simulink model "RLS_mass"  (R2022b)
settings: Solver=VariableStepAuto  StartTime=0.0  StopTime=160  RelTol=1e-3
libraries: ctrlSharedLib x1
settings Model: Creator=EMS0029  LastModifiedBy=EMS0029

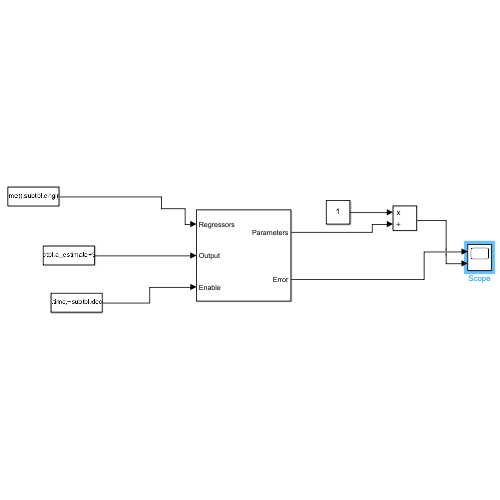
[thumbnail: Simulink's stored preview of the top-level diagram]
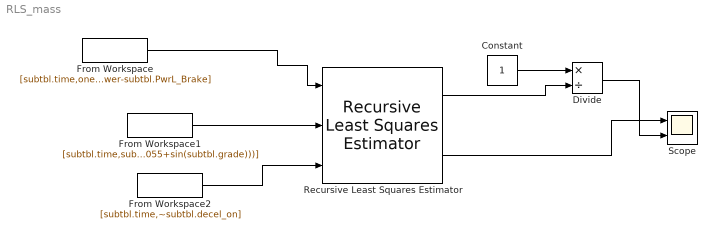
== system RLS_mass ==
  Constant : Constant
  Divide : Product  Inputs=*/
  From Workspace : FromWorkspace  VariableName=[subtbl.time,ones(size(subtbl.time)),subtbl.engine_power-subtbl.PwrL_Brake]  SampleTime=.1
  From Workspace1 : FromWorkspace  VariableName=[subtbl.time,subtbl.v_noise.*(subtbl.a_estimate+9.8*(0.0055+sin(subtbl.grade)))]  SampleTime=.1
  From Workspace2 : FromWorkspace  VariableName=[subtbl.time,~subtbl.decel_on]  SampleTime=.1
  Recursive Least Squares Estimator : ctrlSharedLib/Recursive Least Squares Estimator  InitialEstimateSource=None  InitialParameterData=2  P0=1e8  InitialRegressors=0  InitialOutputs=0  History=Infinite  WindowLength=200  EstimationMethod=Forgetting Factor  AdaptationParameter=.98  HasTimeVaryingAdaptationParameter=off  NormalizationBias=eps  OutputError=on  OutputP=off  AddEnablePort=on  InputProcessing=Sample-based  Ts=-1
      settings: LibrarySourceBlock=slident/Estimators/Recursive Least Squares Estimator
  Scope : Scope  NumInputPorts=2
  wires:
  From Workspace/1 -> Recursive Least Squares Estimator/1
  From Workspace1/1 -> Recursive Least Squares Estimator/2
  Recursive Least Squares Estimator/1 -> Divide/2
  Constant/1 -> Divide/1
  Divide/1 -> Scope/2
  From Workspace2/1 -> Recursive Least Squares Estimator/3
  Recursive Least Squares Estimator/2 -> Scope/1
